simulink model "plant"  (R2021a)
settings: Solver=VariableStepAuto  StartTime=0.0  StopTime=10.0  RelTol=1e-3
model workspace (MATLAB code in the model file):
  | %% Paramètres
  | 
  | g = 10;
  | alpha = 1;
  | l = .8;
  | 
  | %% Valeurs d'équilibre
  | 
  | ubar = 0;
  | dbar = 0;
  | xbar = -(ubar + dbar)/g;
  | vbar = 0;
  | thetabar = 0;
  | qbar = 0;
  | 
  | statebar = [xbar; vbar; thetabar; qbar];
libraries: simulink x2
settings Model: Creator=david  LastModifiedBy=david

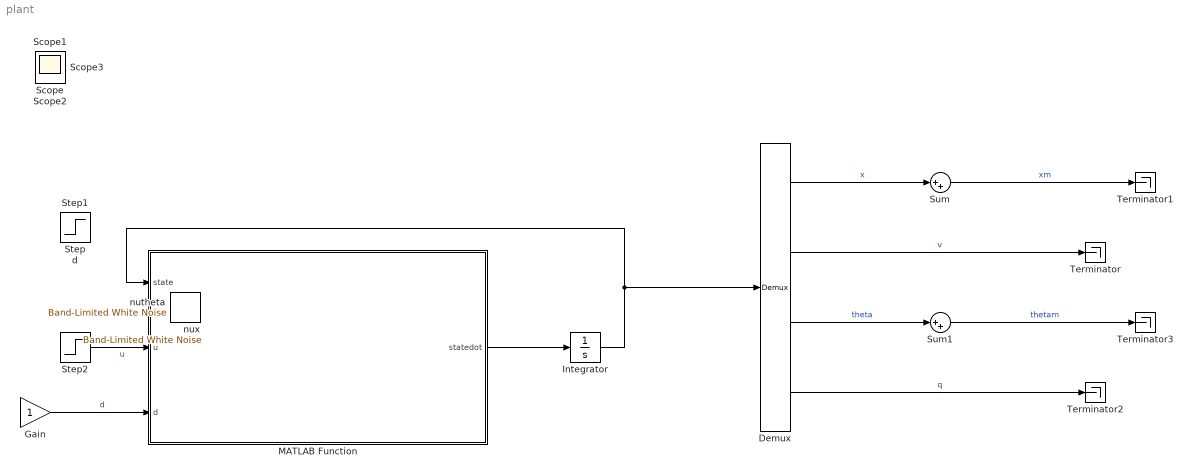
== system plant ==
  Demux : Demux
  Gain : Gain
  Integrator : Integrator  InitialCondition=statebar
  MATLAB Function : MATLAB Function  TreatAsAtomicUnit=on
  Step2 : Step  Before=ubar  After=ubar + .01  SampleTime=0
  Sum : Sum  Inputs=|++
  Sum1 : Sum  Inputs=|++
  Terminator{,1..3} (4 alike) : Terminator
  Scope{,1..3} (4 alike) : Scope
  Step : Step  IOType=siggen  SampleTime=0
  Step1 : Step  IOType=siggen  SampleTime=0
  d : Step  IOType=siggen  Time=2.5  Before=dbar  After=dbar  SampleTime=0
  nutheta : simulink/Sources/Band-Limited White Noise  IOType=siggen  Cov=1e-8  Ts=1e-2  seed=20
  nux : simulink/Sources/Band-Limited White Noise  IOType=siggen  Cov=1e-8  Ts=1e-2  seed=10
  wires:
  MATLAB Function/1(statedot) -> Integrator/1
  Integrator/1 -> MATLAB Function/1(state), Demux/1
  Step2/1 -> MATLAB Function/2(u)  "u"
  Gain/1 -> MATLAB Function/3(d)  "d"
  Demux/2 -> Terminator/1  "v"
  Demux/1 -> Sum/1  "x"
  Sum/1 -> Terminator1/1  "xm"
  Demux/4 -> Terminator2/1  "q"
  Demux/3 -> Sum1/1  "theta"
  Sum1/1 -> Terminator3/1  "thetam"

== matlab function plant/MATLAB Function ==
  data: state input; statedot output; u input; d input; alpha parameter; g parameter
function statedot = fcn(state, u, d, alpha, g)
% Paramètres : alpha = J/m et g, constante de pesanteur terrestre

% Variables d'état
x = state(1);
v = state(2);
theta = state(3);
q = state(4);

% Équations du système
xdot = v;
vdot = x*q^2 + g*sin(theta);
thetadot = q;
qdot = (g*x*cos(theta) + u + d - 2*x*q*v)/(alpha + x^2);

% Output
statedot = [xdot; vdot; thetadot; qdot];
